simulink model "Line_transform_error"  (R2017b)
settings: Solver=VariableStepAuto  StartTime=0.0  StopTime=10.0  RelTol=1e-3
settings Model: Creator=Jesus  LastModifiedBy=Jesus

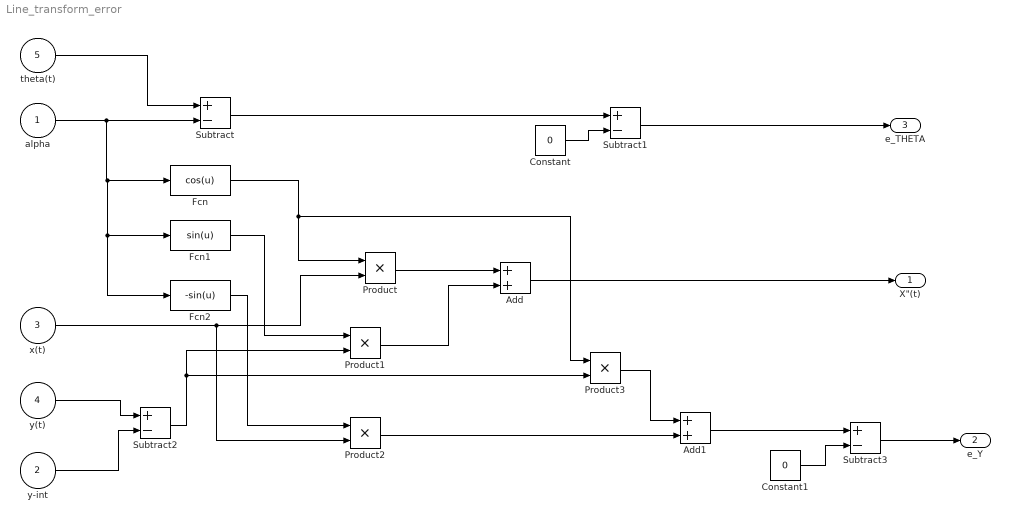
== system Line_transform_error ==
  "alpha " : Inport
  "y-int " : Inport  Port=2
  "x(t) " : Inport  Port=3
  y(t) : Inport  Port=4
  "theta(t) " : Inport  Port=5
  Add : Sum
  Add1 : Sum
  Constant : Constant  Value=0
  Constant1 : Constant  Value=0
  Fcn : Fcn  Expr=cos(u)
  Fcn1 : Fcn  Expr=sin(u)
  Fcn2 : Fcn  Expr=-sin(u)
  Product{,1..3} (4 alike) : Product
  Subtract{,1..3} (4 alike) : Sum  Inputs=+-
  "X\"(t) " : Outport
  "e_Y " : Outport  Port=2
  e_THETA : Outport  Port=3
  wires:
  "theta(t) "/1 -> Subtract/1
  Subtract/1 -> Subtract1/1
  Constant/1 -> Subtract1/2
  Subtract1/1 -> e_THETA/1
  "alpha "/1 -> Fcn2/1, Fcn1/1, Fcn/1, Subtract/2
  "x(t) "/1 -> Product/2, Product2/2
  Product/1 -> Add/1
  y(t)/1 -> Subtract2/1
  "y-int "/1 -> Subtract2/2
  Subtract2/1 -> Product3/2, Product1/2
  Fcn1/1 -> Product1/1
  Product1/1 -> Add/2
  Add/1 -> "X\"(t) "/1
  Fcn2/1 -> Product2/1
  Product2/1 -> Add1/2
  Fcn/1 -> Product3/1, Product/1
  Product3/1 -> Add1/1
  Add1/1 -> Subtract3/1
  Constant1/1 -> Subtract3/2
  Subtract3/1 -> "e_Y "/1
